simulink model "multi_stage"  (Simulink 7.0)
settings: Solver=ode45  StartTime=0.0  StopTime=24/3000  RelTol=1e-6
PreLoadFcn:
  | load one_stage.mat
  | load multi_stage.mat
undefined symbols (not defined in the file or in its folder): hm
libraries: dspmlti4 x4, simulink_extras x2, simulink x2
(part 2 of 2)

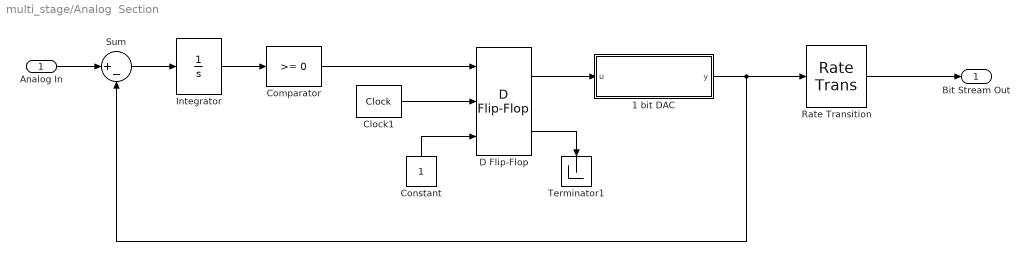
== system multi_stage/Analog  Section ==
  Analog In : Inport  OutDataType=sfix(16)  OutScaling=2^0
  1 bit DAC : Stateflow chart
  Clock1 : simulink_extras/Flip Flops/Clock  SystemSampleTime=-1  MaskParam1=1/(48e3*64)
  Comparator : simulink/Logic and Bit Operations/Compare To Zero  SystemSampleTime=-1  relop=>=  LogicOutDataTypeMode=boolean  ZeroCross=off
  Constant : Constant  Orientation=up  OutDataType=sfix(16)  OutScaling=2^0  SampleTime=0
  D Flip-Flop : simulink_extras/Flip Flops/D Flip-Flop  SystemSampleTime=-1
  Integrator : Integrator
  Rate Transition : RateTransition  OutPortSampleTime=1/(48e3*64)
  Sum : Sum  Inputs=|+-  OutDataType=sfix(16)  OutScaling=2^0
  Terminator1 : Terminator
      settings: Orientation=down
  Bit Stream Out : Outport  DataType=double  OutDataType=sfix(16)  OutScaling=2^0
  wires:
  Sum/1 -> Integrator/1
  Integrator/1 -> Comparator/1
  Comparator/1 -> D Flip-Flop/1
  Analog In/1 -> Sum/1
  D Flip-Flop/2 -> Terminator1/1
  Clock1/1 -> D Flip-Flop/2
  D Flip-Flop/1 -> 1 bit DAC/1(u)
  Constant/1 -> D Flip-Flop/3
  1 bit DAC/1(y) -> Sum/2, Rate Transition/1
  Rate Transition/1 -> Bit Stream Out/1

== matlab function Analog Section/1 bit DAC ==
  data: u input inherited; y output inherited
function y = DAC_1_bit(u)
% This block supports an embeddable subset of the MATLAB language.
% See the help menu for details.

% This code converts boolean input to a bipolar output (double precision).
% We chose to write this in EML function block but we could have also done 
% this with simulink blocks.

y=-1+2*u;
